simulink model "AirRefueling_Platform_PBVS"  (R2022b)
settings: Solver=ode4  StartTime=0.0  StopTime=60  FixedStep=0.01  RelTol=1e-5  AbsTol=1e-4  EnableMultiTasking=on
InitFcn:
  | F16_Init
values from neighbouring files (symbols this model uses):
  airSpeed = 393.72    [F16_Init.m]
  alpha0 = trimAlpha*180/pi    (= 6.62393794015)    [F16_Init.m]
  altitude = 9843    [F16_Init.m]
  b_ref = 30.0    (= 30)    [F16_Init.m]
  C = [ 1,0,0,zeros(1,15) ... (first row only)    [F16_Init.m]
  C2m = [C(1,:) ... (first row only)    [F16_Init.m]
  Cdr_ = 0.8    [hose_parameter4dock.mat]
  d_cam_rc = [4.7;0.54;-1.45] - [0;0;2.05]    [F16_Init.m]
  d_f_rc = [4.45;0;-3.81]    [F16_Init.m]
  d_pr_cam = d_pr_rc - d_cam_rc    [F16_Init.m]
  d_pr_rc = [8.2;0.45;-3.3]    [F16_Init.m]
  dLEF = 0    [F16_Init.m]
  dtheta10 = [0 0 0 0 0 0 0 0 0 0]    [hose_parameter4dock.mat]
  dtheta20 = [0 0 0 0 0 0 0 0 0 0]    [hose_parameter4dock.mat]
  fi_flag = 1    [F16_Init.m]
  height = 3000    [hose_parameter4dock.mat]
  k_reel = 0.5    [hose_parameter4dock.mat]
  Kc = [ ... (first row only)    [F16_Init.m]
  kd = 500    [hose_parameter4dock.mat]
  Ki = zeros(4,3)    [F16_Init.m]
  Kp = zeros(4,18)    [F16_Init.m]
  l0 = 1.44444444444    [hose_parameter4dock.mat]
  l1 = 2    [hose_parameter4dock.mat]
  l_density = 4.1    [hose_parameter4dock.mat]
  m0 = 5.92222222222    [hose_parameter4dock.mat]
  mass = 636.94    [F16_Init.m]
  Mdr = 29.5    [hose_parameter4dock.mat]
  N = 10    [hose_parameter4dock.mat]
  p0_rc = [-30.7;1;10]    [F16_Init.m]
  Rdr = 0.305    [hose_parameter4dock.mat]
  Rl = 0.0336    [hose_parameter4dock.mat]
  T_reel_initial = 1610    [hose_parameter4dock.mat]
  theta10 = [0.459903280115 0.432776206681 0.412025416789 0.390288667864 0.365355881715 0.340009787283 0.310854701374 0.281345523746 0.248396428993 0.214590627751]    [hose_parameter4dock.mat]
  theta20 = [0 0 0 0 0 0 0 0 0 0]    [hose_parameter4dock.mat]
  trim_ail = 0.00874607850103852    (= 0.00874607850104)    [F16_Init.m]
  trim_control = [trim_thrust;trim_ele;trim_ail;trim_rud]    [F16_Init.m]
  trim_ele = -2.97973164860638    (= -2.97973164861)    [F16_Init.m]
  trim_rud = 0.0680302158182712    (= 0.0680302158183)    [F16_Init.m]
  trim_state1 = [trim_state;0;0;0;0;0;0]    [F16_Init.m]
  trim_thrust = 2279.08519954656    (= 2279.08519955)    [F16_Init.m]
  visual_err = [0;0;0]    [F16_Init.m]
  vt0 = [120 0 0]    [hose_parameter4dock.mat]
undefined symbols (not defined in the file or in its folder): dockingPoint, F, MIL, STD
libraries: etargetslib x11, dspnetwork x10, aerolibconvert2 x6, aerolibasang x4, simulink x2, aerolibatmos2 x2, aerolibwind2 x2, aerolibobsolete x2, sharedtransform x2, aerolibutil x2, vrlib x1, aerolibadyn x1
(part 3 of 3)

== matlab function AirRefueling_Platform_PBVS/Hose-drogue system/MATLAB Function ==
  data: P_dr input; P_link10 input; P_hose_dr output
function P_hose_dr = fcn(P_dr,P_link10)
% P_link20=zeros(3,20);
% P_link20(:,1) = P_link10(:,1)/2;
% P_link20(:,2) = P_link10(:,1);
% P_link20(:,3) = (P_link10(:,2)+P_link10(:,1))/2;
% P_link20(:,4) = P_link10(:,2);
% P_link20(:,5) = (P_link10(:,3)+P_link10(:,2))/2;
% P_link20(:,6) = P_link10(:,3);
% P_link20(:,7) = (P_link10(:,4)+P_link10(:,3))/2;
% P_link20(:,8) = P_link10(:,4);
% P_link20(:,9) = (P_link10(:,5)+P_link10(:,4))/2;
% P_link20(:,10) = P_link10(:,5);
% P_link20(:,11) = (P_link10(:,6)+P_link10(:,5))/2;
% P_link20(:,12) = P_link10(:,6);
% P_link20(:,13) = (P_link10(:,7)+P_link10(:,6))/2;
% P_link20(:,14) = P_link10(:,7);
% P_link20(:,15) = (P_link10(:,8)+P_link10(:,7))/2;
% P_link20(:,16) = P_link10(:,8);
% P_link20(:,17) = (P_link10(:,9)+P_link10(:,8))/2;
% P_link20(:,18) = P_link10(:,9);
% P_link20(:,19) = (P_link10(:,10)+P_link10(:,9))/2;
% P_link20(:,20) = P_link10(:,10);
% %P_link20(:,20) = P_dr;
% P_link20_V60 = reshape(P_link20,60,1);


%% 

x = P_link10(1,:);
y = P_link10(2,:);
z = P_link10(3,:);
n=length(x)-1;% B样条曲线有n+1个控制点
k=4;% 三次B样条，因此阶数=次数+1

% 用于储存生成的点
X=[];
Y=[];
Z=[];

Nik_u=zeros(1,n+1);% 用于储存基函数
nodevector=U_quasi_uniform(n,k);% 生成节点向量

for u=0:0.01:1-0.01% 循环次数决定组成B样条曲线点的总数量
    for j=1:n+1% 生成Bi,3这一系列基函数
        Nik_u(j)=BaseFunction(j,k,u,nodevector);
    end
    % 由于B样条曲线具有局部支撑性，因此只有u周围一定区间会参与到计算
    X=[X,x*Nik_u'];
    Y=[Y,y*Nik_u'];
    Z=[Z,z*Nik_u'];
end
% 根据三次B样条插值的结果得到20根管子的位置
P_link20=zeros(3,20);
index = 1;
for i=1:length(X)/20:100
    P_link20(:,index)=[X(i),Y(i),Z(i)];
    index = index+1;
end

P_link20_V60 = reshape(P_link20,60,1);
% 再将锥套的真实位置传过去 此时是63*1(20根管子+1个锥套)的向量 前面60个是软管 最后三个是锥套
P_hose_dr = [P_link20_V60;P_dr];

== matlab function AirRefueling_Platform_PBVS/Hose-drogue system/DRdynamics/Hose-Drogue1/Calculate the External Force of the Links/MATLAB Function ==
  data: vr input; n input; Ref output; radius input; viscosity input; Cf output; Red output; Cd output; N parameter
function [Ref, Cf, Red, Cd] = C(vr,n,radius,viscosity, N)
% 计算雷诺数以及相应的摩擦系数Cf和压差系数Cd

% 单杆的速度、方向等用3*1的列向量表示
% vr = 连杆相对风速度 向量3*N
% n = 连杆的方向向量，想上为正 向量3*N
% viscosity  = 动粘度系数
% radius = 连杆半径

%——计算雷诺数———————————————————————————
cosa = zeros(1,N);
sina = zeros(1,N);
Ref = zeros(1,N);
Red = zeros(1,N);
for i = 1:N
    if norm(vr(:,i)) ~= 0
        cosa(i) = vr(:,i)'*n(:,i)/norm(vr(:,i));
        sina(i) = sqrt(1-cosa(i)^2);
        if sina(i) ~= 0
            Ref(i) = (pi*radius/viscosity)*norm(vr(:,i))/sina(i);
        else
            Ref(i) = 10^11;
        end
        Red(i) = norm(vr(:,i))*2*radius/viscosity;
    end
end

%——计算气动系数——————————————————————————
Cf = zeros(1,N);
Cd = zeros(1,N);
for i = 1:N
    %%%%Cf表%%%%%%%%%%%%%%%%%%%%%%%%
    if Ref(i)<=10^-2
        Cf(i) = 0;    %注意这里有改动
    elseif Ref(i)>10^-2 && Ref(i)<=10^4
        Cf(i) = 4.6409*Ref(i)^-0.6667;
    elseif Ref(i)>10^4 && Ref(i)<=10^10
        Cf(i) = 0.0464*Ref(i)^-0.1667;
    elseif Ref(i)>10^10
        Cf(i) = 0.001;
    end
    %%%%Cd表%%%%%%%%%%%%%%%%%%%%%%%%%
    if Red(i)<=10^-2
        Cd(i) = 0;   %注意这里有改动
    elseif Red(i)>10^-2 && Red(i)<=1
        Cd(i) = 10*Red(i)^-0.801;
    elseif Red(i)>1 && Red(i)<=180
        Cd(i) = 10*Red(i)^-0.4083;
    elseif Red(i)>180 && Red(i)<=4*10^5
        Cd(i) = 1.2;
    elseif Red(i)>4*10^5 && Red(i)<=4*10^6
        Cd(i) = 0.002128*Red(i)^0.3522;
    elseif Red(i)>4*10^6
        Cd(i) = 0.45;
    end
end

== matlab function AirRefueling_Platform_PBVS/Hose-drogue system/DRdynamics/Hose-Drogue1/Calculate the External Force of the Links/MATLAB Function1 ==
  data: vr input; Q output; n input; Cf input; Cd input; l1 input; density input; radius input; Rdr input; Cdr input; Mdr input; rou input; p input; Fb input; Df_mid output; Dd_mid output; Df output; Dd output; D output; Ddr output; N parameter; l0 parameter; fen_norm output; fen output
function [Q, Df_mid, Dd_mid, Df, Dd, D, Ddr, fen_norm, fen] = ExternalForce(vr,n,Cf,Cd,l1,density,radius,Rdr,Cdr,Mdr,rou,p,Fb, N,l0)

% 计算每根连杆的合外力

% 单杆的速度、方向等用3*1的列向量表示
% l = 每根连杆的长度，注意这里要做成变长的 向量
% vr = 连杆相对风速度 向量3*N
% n = 连杆的方向向量，想上为正 向量3*N
% viscosity  = 大气动粘度系数
% density = 大气密度
% radius = 连杆半径
% r_dr = 锥套伞冠半径
% rou = 连杆的线密度

% Cdr = 锥套的阻力系数
% Rdr = 锥套伞冠半径
% Mdr = 锥套质量

%——求气动力————————————————————————————
Df_mid = zeros(1,N);
Dd_mid = zeros(1,N);
Df = zeros(3,N);
Dd = zeros(3,N);
D = zeros(3,N);
vn = zeros(3,N);
for i = 1:N
    if i == 1
        Df_mid(i) = density*pi*radius*l1*Cf(i)*(vr(:,i)'*n(:,i))^2;
    else
        Df_mid(i) = density*pi*radius*l0*Cf(i)*(vr(:,i)'*n(:,i))^2;
    end
    if vr(:,i)'*n(:,i)>0   % 这里可能有符号问题，万一之后还是出现杂乱的情况，要注意这里
        Df(:,i) = Df_mid(i)*n(:,i);
    else
        Df(:,i) = - Df_mid(i)*n(:,i);
    end
    % 当杆的方向迎着风的时候，摩擦阻力延杆反向
    % 当杆的方向顺着风的时候，摩擦阻力延杆正向
    
    vn(:,i) = vr(:,i)-(vr(:,i)'*n(:,i))*n(:,i); 
    if i == 1
        if norm(vn(:,i)) ~= 0
            Dd_mid(i) = density*radius*l1*Cd(i)*norm(vn(:,i))^2;
            Dd(:,i) = - Dd_mid(i)*vn(:,i)/norm(vn(:,i));
        else
            Dd(:,i) = [0;0;0];
        end
    else
        if norm(vn(:,i)) ~= 0
            Dd_mid(i) = density*radius*l0*Cd(i)*norm(vn(:,i))^2;
            Dd(:,i) = - Dd_mid(i)*vn(:,i)/norm(vn(:,i));
        else
            Dd(:,i) = [0;0;0];
        end
    end
    % 无论连杆与相对速度的角度关系如何，压差阻力总是顺着风的方向的
        
    D(:,i) = Df(:,i) + Dd(:,i);
end

if vr(:,N)'*vr(:,N) ~= 0
    Ddr = - 1/2*density*vr(:,N)'*vr(:,N)*(pi*Rdr^2)*(Cdr)* vr(:,N)/norm(vr(:,N));
else
    Ddr = [0;0;0];
end
%%%%%%%%%%%%%%%%%%%%%%%%%%%%%%%%%%%%%%%%%%%%%%%%%%%%%%%%%%%%%%%%

% %%%%计算恢复力%%%%%%%%%%%%%%%%%%%%%%
do = 1; % 连杆外径
di = 0.84; % 连杆内径
E = 589.67; % 弹性系数 数量级可能有问题
K = E*pi/8*(do^4 - di^4);
fen_norm = zeros(1,N);
fen = zeros(3,N);
for i = 2:N-1
    n0mid = (p(:,i-1) - p(:,i+1))/norm(p(:,i-1) - p(:,i+1));
    if abs(norm(n(:,i-1)'*n(:,i))-1) ~= 0;
        gama1 = n(:,i-1)'*n0mid;
        gama2 = n(:,i)'*n0mid;
        if norm(gama1) >= 1
            gama1 = gama1/abs(gama1);
        end
        if norm(gama2) >= 1
            gama2 = gama2/abs(gama2);
        end
            
        fen_norm(i) = K*(acos(gama1) + acos(gama2))/norm(p(:,i-1) - p(:,i+1))^2;
        fen(:,i) = fen_norm(i)*((n(:,i)'*n0mid*n0mid - n(:,i))*1e3)/norm((n(:,i)'*n0mid*n0mid - n(:,i))*1e3);
    end
end
%%%%%%%%%%%%%%%%%%%%%%%%%%%%%%%%%%%%%%

% %%%%计算合外力%%%%%%%%%%%%%%%%%%%%%%?
% Q = zeros(3,N);
% for i = 1:N-1
%     Q(:,i) = [0;0;m*g] + 1/2*(D(:,i)+D(:,i+1));
% end
% Q(:,N) = [0;0;(m+Mdr)*g] + 1/2*D(:,N) + Ddr;
Q = zeros(3,N);
Q(:,1) = [0;0;l1*rou*9.8] + 1/2*(D(:,1)+D(:,2)) + fen(:,1);
for i = 2:N-1
    Q(:,i) = [0;0;l0*rou*9.8] + 1/2*(D(:,i)+D(:,i+1)) + fen(:,i);
end
Q(:,N) = [0;0;(l0/2*rou + Mdr)*9.8] + 1/2*D(:,N) + Ddr + Fb;        %注意最后一个节点的质量
% 这里删掉了锥套的受力（Bow wave），后面再处理
% %%%%%%%%%%%%%%%%%%%%%%%%%%%%%%%%

== matlab function AirRefueling_Platform_PBVS/Hose-drogue system/DRdynamics/Hose-Drogue1/Calculate the Orientation of the Links1/MATLAB Function ==
  data: nd1 output; nd2 output; theta1 input; n output; theta2 input; N parameter
function [nd1,nd2,n] = fcn(theta1,theta2, N)
% theta1,theta2 向量1*n
n = zeros(3,N);
nd1 = zeros(3,N);
nd2 = zeros(3,N);

for i = 1:N
    n(:,i) = [cos(theta1(i))*cos(theta2(i)); sin(theta2(i)); -sin(theta1(i))*cos(theta2(i))];
    nd1(:,i) = [-sin(theta1(i))*cos(theta2(i)); 0; -cos(theta1(i))*cos(theta2(i))];
    nd2(:,i) = [-cos(theta1(i))*sin(theta2(i)); cos(theta2(i)); sin(theta1(i))*sin(theta2(i))];
end

== matlab function AirRefueling_Platform_PBVS/Hose-drogue system/DRdynamics/Hose-Drogue1/Calculate the Orientation of the Links1/MATLAB Function4 ==
  data: a input; a0 input; nd1 input; nd2 input; dn input; dnd1 input; dnd2 input; dtheta1 input; dtheta2 input; l1 input size=1; dl1 input; ddtheta1 output; ddtheta2 output; N parameter; l0 parameter
function [ddtheta1,ddtheta2] = fcn(a,a0,nd1,nd2,dn,dnd1,dnd2,dtheta1,dtheta2,l1,dl1, N, l0)
% theta1,theta2 向量N*1
% omiga,alpha是加油机坐标系的旋转角速度和叫加速度
% a是各节点的加速度
% a0为加油机加速度
% l,dl,ddl是连杆的长度及其一二阶导数

ddtheta1 = zeros(1,N);
ddtheta2 = zeros(1,N);

ddtheta1(1) = nd1(:,1)'*(-(a(:,1)-a0)-2*dl1*dn(:,1)-...
              l1*(dnd1(:,1)*dtheta1(1)+dnd2(:,1)*dtheta2(1)))...
              /(l1*norm(nd1(:,1)));
ddtheta2(1) = nd2(:,1)'*(-(a(:,1)-a0)-2*dl1*dn(:,1)-...
              l1*(dnd1(:,1)*dtheta1(1)+dnd2(:,1)*dtheta2(1)))...
              /(l1*norm(nd2(:,1)));
for i = 2:N
    ddtheta1(i) = nd1(:,i)'*(-(a(:,i)-a(:,i-1))-...
                  l0*(dnd1(:,i)*dtheta1(i)+dnd2(:,i)*dtheta2(i)))...
                  /(l0*norm(nd1(:,i)));
    ddtheta2(i) = nd2(:,i)'*(-(a(:,i)-a(:,i-1))-...
                  l0*(dnd1(:,i)*dtheta1(i)+dnd2(:,i)*dtheta2(i)))...
                  /(l0*norm(nd2(:,i)));
end

== matlab function AirRefueling_Platform_PBVS/Hose-drogue system/DRdynamics/Hose-Drogue1/Calculate the Orientation of the Links1/MATLAB Function5 ==
  data: v0 input; n input; dn input; l1 input; dl1 input; w input; vr output; p0 input; p output; N parameter; l0 parameter; pdr output
function [vr,p,pdr] = fcn(v0,n,dn,l1,dl1,w,p0, N, l0)

% v0为加油机速度
% l,dl是连杆的长度及其一阶导数
% wt为合成风在每个节点的风速
% p0为预留，在计算相对地面的位置时用到

vr = zeros(3,N);
vr(:,1) = v0 - dl1*n(:,1) - l1*dn(:,1) ;
for i = 2:N
    vr(:,i) = vr(:,i-1) - l0*dn(:,i);
end
vr = vr - w;

p = zeros(3,N);
p(:,1) = [0;0;0] - l1*n(:,1);
for i = 2:N
    p(:,i) = p(:,i-1) - l0*n(:,i);
end
pdr = p(:,N) + [-0.3;0;0];
% pdr = p(:,N);

== matlab function AirRefueling_Platform_PBVS/Receiver system/Guidance ==
  settings: updateMethod=DISCRETE
  data: dd input; estimate_dr2pr input; y output; t input; d_x output; t_d output
function [y,d_x,t_d] = fcn(dd,estimate_dr2pr,t)
%#codegen
%dd是锥管前端位置，dx是锥套位置（dx输入前第三分量换号，已由x,y,h转化为x,y,z）
%dx输入前减去常数：控制中控制的是受油机质心而非锥管前端，所以参考轨迹也要由锥管的参考轨迹转化为受油机质心的参考轨迹。
%控制的目的就是最终令dd和dx相等，让受油机质心跟踪参考位置

% y=dx; 输出y的意思是让受油机飞行的三维距离，和之前初始化定义受油机三维位置不同
%% 理想的对接点是  [9.5100;-1.4550;-0.0830]+[0.2;0;0] 9.5m时是第一节探头进锥套 最多再多0.2m此时是第一节抵住中间小黑圈
persistent aa;
if(isempty(aa))   %%aa(1:3)为锥套平衡位置,(4:6)为锥套实际位置或其滤波位置，(7:9)是锥管实际位置或其滤波位置；
    aa=zeros(9,1);
end

% 这个tt是用来对总体的时间逻辑进行控制的
persistent tt;
if(isempty(tt))
    tt=0;
end
% 这个t_dock是用来记录对接成功的初始时间的，这样就能
persistent t_dock;
if(isempty(t_dock))
    t_dock=0;
end
t_d=t_dock;

% 这个t_lock是用来锁定对接时间的，标识为1时说明已经锁定了对接时间
persistent t_lock;
if(isempty(t_lock))
    t_lock=0;
end

% 判断是否可以脱离对接，再进行下一次的对接
persistent flag_can_dock;
if(isempty(flag_can_dock))
    flag_can_dock=1;
end

persistent nn;    %%nn为前馈量
if(isempty(nn))
    nn=[0;0;0];
end

persistent dx;     %%锥套位置距离其平衡位置的偏差
if(isempty(dx))
    dx=[0;0;0];
end
d_x=dx;

% 使用额外飞行的距离来对碰撞模块和HDU进行验证
extra_flight=[0.5;0;0];
%% y为期望轨迹
% tt是上次对接成功时候记录的时间
t1=t-tt;
if t1<20
    y=[8;-1.8;0.4];
    aa(1:3)=y;
elseif t1<30
    y = aa(1:3);
    if t1>24 && t1<25
        % 此时的aa(1:3)约等于[8;-1.8;0.4]，estimate_pr2dt=[1.61;0.345;-0.483]
        dx = aa(1:3)+ estimate_dr2pr;
    end
    if t1>25
        dx(1:3) = 3/4 * dx(1:3) + 1/4 * (aa(1:3) + estimate_dr2pr);
    end
else   
    y = [dx(1)+nn(1);dx(2)+nn(2);dx(3)+nn(3)]+extra_flight ; 
%     y = 0.5 * ([dx(1)+nn(1);dx(2)+nn(2);dx(3)+nn(3)]+[dx(1)+dd(1);dx(2)+dd(2);dx(3)+dd(3)]);     
%%  这里是近距离对接过程的判断
    if abs(dd(1)-dx(1))<0.01 && flag_can_dock == 1  % 状态为可以对接 且 锥管锥套距离达到对接要求 认为是一次对接
       % 认为已经对接上了 所以标志位要清零, 同时记录对接的时间t_dock
       flag_can_dock = 0;
       t_lock = 1;
       if(t_lock == 1 && flag_can_dock == 0)
           % 在对接成功时，虽然满足0.01的条件，但是不满足后面==1的条件 所以对接时间不会多次记录
          t_dock = t;
       end
    end
    
   % t_dock保存的就是对接成功的时间 当保持的时间大于20s时，才进行下一次对接
   % 在对接状态 且 持续时间超过了10s 就设置为脱离状态
   if(t-t_dock>=10 && flag_can_dock == 0 )
       flag_can_dock=1;
           % 如果对接的时间到 那么锥套椎管放开接触 标志位置1，意味着可以对接
       if(flag_can_dock == 1)
           % 更新前馈量 aa(4:6)存储的是锥套的滤波位置 aa(7:9)存储的是椎管的滤波位置
           nn=nn+[0.6*sat((aa(4)-aa(7))/0.6);0.6*sat((aa(5)-aa(8))/0.6);0.6*sat((aa(6)-aa(9))/0.6)];

           % 省去了前面的过程  时间如果一减掉 调用脚本的时候就跳出这个代码范围 相当于回到第10s时候的状态
           tt=t-10;
       end   
   end    
          
    % 当距离小于0.4m的时候，进行滤波
    if abs(dd(1)-dx(1))<0.4 && flag_can_dock == 1
        aa(4:6)=2/3 * aa(4:6)+ 1/3 * dx;
        aa(7:9)=2/3 * aa(7:9)+ 1/3 * dd;
    end  
    % 当小于0.5m大于0.4m的时候，记录位置
    if abs(dd(1)-dx(1))<0.5 && flag_can_dock == 1
        aa(4:6)=dx;
        aa(7:9)=dd;
    end 
end

== matlab function AirRefueling_Platform_PBVS/Hose-drogue system/DRdynamics/Hose-Drogue1/MATLAB Function3 ==
  data: n input; alpha output; N parameter
function alpha = fcn(n, N)
% 计算两杆之间的弯折角度，用来粗略的验证恢复力的效果
alpha = zeros(1,N);
for i = 2:N
    mid = n(:,i-1)'*n(:,i);
    if abs(mid) > 1
        mid = mid/abs(mid);
    end
    alpha(i) = acos(mid)/pi*180;
end

== matlab function AirRefueling_Platform_PBVS/Visual process/VehicleDataParse ==
  data: Data input; CopterID output; Length input; Out output; checksum input; len input
function [CopterID,Out] = fcn(Data,Length,checksum,len)

% 设定静态变量，在数据校验失败时，保持上一时刻值
persistent DataOut;
if isempty(DataOut)
    DataOut=zeros(16,1);
end
persistent cpID;
if isempty(cpID)
    cpID=0;
end

% 如果包长不等于设定值，这个包丢弃，使用原来的值
if Length ~= len %如果包长度不匹配，校验不通过，那么使用上一时刻值
    Out=DataOut;
    CopterID=cpID;
    return;
end

CkSum = typecast(Data(1:4), 'int32');
if CkSum ~= checksum %如果校验码不匹配，校验不通过，那么使用上一时刻值
    Out=DataOut;
    CopterID=cpID;
    return;    
end

% 提取数据
CpIDTmp = typecast(Data(5:8), 'int32');
DataTmp = typecast(Data(9:136), 'double');
% DataTmp=zeros(16,1);
for i=1:16
    idx = (i-1)*8+9;
    DataTmp(i) = typecast(Data(idx:idx+7), 'double');
end



% 配置输出数据
CopterID = double(CpIDTmp);
Out = DataTmp;

% 记录上一时刻值
cpID=CopterID;
DataOut=Out;

== matlab function AirRefueling_Platform_PBVS/SimToUE11 ==
  data: y output; PosPr1 input; PosTb1 input
function y = SimToVR(PosPr1,PosTb1)
%#codegen

%%函数名：SimToVR
%%用途  ：将软管锥套坐标输出转换为VR输入
%%输入  ：PosPr - 受油机椎管坐标， PlsTb - 软管坐标数据
%%输出  ：VrPos - 软管和受油机VR位置，VrAngle - 旋转角度输出
%%作者  ：戴训华
%%时间  ：2014/3/19

%{
PosPr = PosPr1(1:3);
% add PosPr1(4:6)存储的是受油机的姿态  模型中在输出姿态[phi, theta, psai]后加上了trim_state1=[0;0.1156,0],这里又给减掉了
% 无人机先绕机体系 z 轴旋转 ψ \psiψ，再绕机体系 y 轴旋转 θ \thetaθ，最后绕机体系 x 轴旋转 ϕ \phiϕ，[yaw,pitch,roll]
% AttitudeRecei = [PosPr1(4);-PosPr1(6);PosPr1(5)-0.115609];
AttitudeRecei = [PosPr1(4);-PosPr1(6);PosPr1(5)-0.115609];
PosTb = PosTb1(1:60);
% 这里是20根软管+1个锥套+1个受油机 
VrAngle = zeros(22*3,1);
VrPos = zeros(22*3,1);
% add
scale = 1;
for j = 1:21                        %前20为软管坐标数据，后1为软管平滑过渡处理
    if j == 1
        pX = [0, 0, 0]';            %软管起点
        pY = PosTb(3*j-2:3*j);      %软杆终点
    elseif j == 21                  %多加一段杆，做过渡
        pX = PosTb(3*j-5:3*j-3);
        pY = [PosTb(3*j-5)-0.7163*cos(8/180*pi),PosTb(3*j-4),PosTb(3*j-3)+0.7163*sin(8/180*pi)]';
    else
        pX = PosTb(3*j-5:3*j-3);
        pY = PosTb(3*j-2:3*j); 
    end
    
    pZ = (pX + pY)/2;               %中点坐标
    if j==21
        % 给一个锥套的偏置
        pZ = pZ + [0,0,-0.25]';
    end
%     pZ = pZ * 8/3;                  %到VR中比例的缩放
    pZ = pZ * scale;
    
    vAxis = [0,0,-1]';               %水平轴
    vTb = pY - pX;                  %杆的方向
    
    axis1 = null([vAxis';vTb']);%获取垂直向量
    vRot = axis1(:,1)';             %得到旋转轴
    
    if vRot(2) < 0
        vRot = -vRot;
    end
 
    yaw_xoz = asin(vTb(2) / sqrt(vTb(1)*vTb(1) + vTb(2)*vTb(2)+ vTb(3)*vTb(3)));
    pitch_z = pi - atan(vTb(3) / vTb(1));
%     pitch_z = atan(vTb(3) / vTb(1));
    roll = 0;   % 圆柱形hose，不用计算roll   
    VrAngle(3*j-2:3*j) = [yaw_xoz, pitch_z, roll];
    VrPos(3*j-2:3*j) = [pZ(1),pZ(2),pZ(3)]';
end
%y = u;
% add 发送的是受油机的位置
VrAngle(64:66)=[AttitudeRecei(1);AttitudeRecei(2);AttitudeRecei(3)];
% add PosPr(1:3)受油机椎管的坐标  [0 -0.1 -0.05]'是椎管相对于受油机的位置
pZ = PosPr+[0 -0.1 -0.05]';
pZ = pZ * scale;
% pZ = pZ * 8/3;
% 旋转坐标系
VrPos(3*22-2:3*22) = [pZ(1),pZ(2),pZ(3)]';
tmp1 = VrPos(1:60,:); % 软管位置
% delta_drogue =[0 0 0.5]'; 
delta_drogue =[-0.8 0 0.45]'; 
% delta_drogue =[-0.2 0 0.3]'; 
tmp2 = VrPos(61:63,:)+ delta_drogue;% 锥套位置
tmp3 = VrPos(64:66,:);% 受油机位置
tmp4 = VrAngle(1:60,:); % 软管角度
tmp5 = VrAngle(61:63,:)+[0 0.09 0]';% 锥套角度
tmp6 = VrAngle(64:66,:);% 受油机角度
tmp=[tmp1;tmp4;tmp2;tmp5;tmp3;tmp6];
y = tmp;
%}

%%
%%函数名：SimToVR
%%用途  ：将软管锥套坐标输出转换为VR输入
%%输入  ：PosPr - 受油机椎管坐标， PlsTb - 软管坐标数据 60*1 10根管子的位置（每根管子的中心位置和尾部位置，一共10*3+10*3=60个数据） 
%%输出  ：VrPos - 软管和受油机VR位置，VrAngle - 旋转角度输出

PosPr = PosPr1(1:3);
% add PosPr1(4:6)存储的是受油机的姿态  模型中在输出姿态[phi, theta, psai]后加上了trim_state1=[0;0.1156,0],这里又给减掉了
% 无人机先绕机体系 z 轴旋转 ψ \psiψ，再绕机体系 y 轴旋转 θ \thetaθ，最后绕机体系 x 轴旋转 ϕ \phiϕ，[yaw,pitch,roll]
% AttitudeRecei = [PosPr1(4);-PosPr1(6);PosPr1(5)-0.115609];
% AttitudeRecei = [PosPr1(4);PosPr1(5);PosPr1(6)];
AttitudeRecei = [0;0.1156;0];
%% 这个模型中是10个软管，传入的60*1的数组中，已经包含了杆子中心的坐标
PosTb = PosTb1(1:60);
% 这里是10根软管+1个锥套+1个受油机,全部是列向量
VrAngle = zeros(12*3,1);
VrPos = zeros(12*3,1);
% add
scale = 1;
for j = 1:11                                        %10根为软管坐标数据 第11根为锥套的坐标数据
    if j == 11                                      %多加一段杆，做过渡
        pX = PosTb(6*(j-1)-2:6*(j-1));              %选择最后一个位置作为锥套的pX
        pY = [PosTb(6*(j-1)-2)-0.7163*cos(8/180*pi),PosTb(6*(j-1)-1),PosTb(6*(j-1))+0.7163*sin(8/180*pi)]';     % 这个位置是平滑出来的，用作方向,大概是虚拟的第11根杆的中点
        pZ = pY + [0,0,0]';
    else
        pX = PosTb(6*(j-1)+1:6*(j-1)+3);            %第一根软管的中点，起点是(0,0,0)
        pY = PosTb(6*(j-1)+4:6*(j-1)+6);            %软杆终点
        pZ = pX;                                    %中点坐标，前面的程序中计算过了，直接赋值
    end
    pZ = pZ * scale;
    vAxis = [0,0,-1]';               %水平轴
    vTb = pY - pX;                  %杆的方向
    
    axis1 = null([vAxis';vTb']);%获取垂直向量
    vRot = axis1(:,1)';             %得到旋转轴
    
    if vRot(2) < 0
        vRot = -vRot;
    end
 
    yaw_xoz = asin(vTb(2) / sqrt(vTb(1)*vTb(1) + vTb(2)*vTb(2)+ vTb(3)*vTb(3)));
    pitch_z = pi - atan(vTb(3) / vTb(1));
%     pitch_z = atan(vTb(3) / vTb(1));
    roll = 0;   % 圆柱形hose，不用计算roll   
    VrAngle(3*j-2:3*j) = [yaw_xoz, pitch_z, roll];
    VrPos(3*j-2:3*j) = [pZ(1),pZ(2),pZ(3)]'+[0,0,-1]';
end
%y = u;
% add 发送的是受油机的姿态
VrAngle(34:36)=[AttitudeRecei(1);AttitudeRecei(2);AttitudeRecei(3)];
% add PosPr(1:3)受油机椎管的坐标  [0 -0.1 -0.05]'是微调椎管相对于受油机的位置
pZ = PosPr+[0 -0.1 -0.05]';
pZ = pZ * scale;
VrPos(34:36) = [pZ(1),pZ(2),pZ(3)]';

tmp1 = VrPos(1:30); % 软管位置
% delta_drogue_pos =[-0.8 0 0.45]'; 
% delta_drogue_atti=[0 0.09 0]';
delta_drogue_pos =[0 0 0]'; 
delta_drogue_atti=[0 0.09 0]';
tmp2 = VrPos(31:33)+ delta_drogue_pos;% 锥套位置
tmp3 = VrPos(34:36);% 受油机位置
tmp4 = VrAngle(1:30); % 软管角度
tmp5 = VrAngle(31:33)+delta_drogue_atti;% 锥套角度
tmp6 = VrAngle(34:36);% 受油机角度
tmp=[tmp1;tmp4;tmp2;tmp5;tmp3;tmp6];
y = tmp;

== matlab function AirRefueling_Platform_PBVS/Hose-drogue system/DRdynamics/Hose-Drogue1/Calculate the Acceleration of the Links1/MATLAB Function ==
  data: n input; m1 input; T output; m0 parameter; N parameter
function T = fcn(n,m1, m0,N)

% n = 连杆的方向向量，想上为正 向量3*N
% m = 连杆的质量 向量1*N

%%%%求张力t%%%%%%%%%%%%%%%%%%%%%%%%%%%%%%%%%%%%%%%%%%%%%%%%%%%%%%
T = zeros(N,N);

T(1,1) = 1;
T(1,2) = - n(:,1)'*n(:,2);
T(N,N-1) = -1/m0*n(:,N-1)'*n(:,N);
T(N,N) = 1/m0 + 1/m0;             %注意这里很重要！！

T(2,1) = -1/m1*n(:,1)'*n(:,2);
T(2,2) = 1/m1 + 1/m0;
T(2,3) = -1/m0*n(:,2)'*n(:,3);

for i = 3:N-1
    T(i,i-1) = -1/m0*n(:,i-1)'*n(:,i);
    T(i,i) = 1/m0 + 1/m0;
    T(i,i+1) = -1/m0*n(:,i)'*n(:,i+1);
end

== matlab function AirRefueling_Platform_PBVS/Tanker system/  ==
  data: u input; y output

function y = WindTurFromTank(u)
%#codegen

%横纵向气流角速度等下计算长度
c_lat=4;
c_lon=4;

%两端参考点
u1 = u+[0 ,c_lat ,0]';
u2 = u+[0 ,-c_lat, 0]';

yy1 = TankerVortexWindField(u1);
yy2 = TankerVortexWindField(u2);

%计算x轴向滚转角速度
yp = (yy1(3) - yy2(3))/4/c_lat;

u3=u+[c_lon, 0,0]';
u4=u+[-c_lon ,0,0]';
yy3 = TankerVortexWindField(u3);
yy4 = TankerVortexWindField(u4);

%俯仰角速度计算
yq = -(yy3(3) - yy4(3))/4/c_lon;

%偏航角速度设为0
yr = 0;

%质心处风场计算
y_uvw = TankerVortexWindField(u);


%y = [y_uvw(1);y_uvw(2);y_uvw(3);-yp;-yq;-yr]*0.5;
y = [y_uvw(1);y_uvw(2);y_uvw(3);-yp;-yq;-yr];

== matlab function AirRefueling_Platform_PBVS/SimToVR1 ==
  data: PosPr1 input; PosTb1 input; y output
function y = SimToVR(PosPr1,PosTb1)
%#codegen

%%函数名：SimToVR
%%用途  ：将软管锥套坐标输出转换为VR输入
%%输入  ：PosPr - 受油机椎管坐标， PlsTb - 软管坐标数据
%%输出  ：VrPos - 软管和受油机VR位置，VrAngle - 旋转角度输出
%%作者  ：戴训华
%%时间  ：2014/3/19

PosPr = PosPr1(1:3);
AttitudeRecei = [0;-0;0+0.115609];

PosTb = PosTb1(1:60);

VrAngle = zeros(22*4,1);
VrPos = zeros(22*3,1);


for j = 1:21                        %前20为软管坐标数据，后1为软管平滑过渡处理
    if j == 1
        pX = [0, 0, 0]';            %软管起点
        pY = PosTb(3*j-2:3*j);      %软杆终点
    elseif j == 21                  %多加一段杆，做过渡
        pX = PosTb(3*j-5:3*j-3);
        pY = [PosTb(3*j-5)-0.7163*cos(8/180*pi),PosTb(3*j-4),PosTb(3*j-3)+0.7163*sin(8/180*pi)]'+[0;-0.2;0];
    else
        pX = PosTb(3*j-5:3*j-3);
        pY = PosTb(3*j-2:3*j); 
    end
    
    pZ = (pX + pY)/2;               %中点坐标
    pZ = pZ * 8/3;                  %到VR中比例的缩放

    vAxis = [0,0,-1]';               %水平轴
    vTb = pY - pX;                  %杆的方向
    
    axis1 = null([vAxis';vTb']);%获取垂直向量
    vRot = axis1(:,1)';             %得到旋转轴
    
    if vRot(2) < 0
        vRot = -vRot;
    end
    
    VrAngle(4*j-3:4*j-1) = [vRot(1),vRot(3),vRot(2)]';
    VrAngle(4*j) = acos(vAxis'*vTb / sqrt(vAxis'*vAxis * vTb'*vTb));
    
    VrPos(3*j-2:3*j) = [pZ(1),-pZ(3),pZ(2)]';
end
%y = u;
VrAngle(81:84)=VrAngle(81:84)+[0.2714;0;0;0]; %微调锥套姿态
VrPos(61:63)=VrPos(61:63)+[0;0.00;0.25];      %微调锥套位置

VrAngle(85:88)=[AttitudeRecei(1);AttitudeRecei(2);AttitudeRecei(3);norm(AttitudeRecei)];
pZ = PosPr+[0 0-0.1 0-0.1]';
pZ = pZ * 8/3;
VrPos(3*22-2:3*22) = [pZ(1),-pZ(3),pZ(2)]';

y = [VrAngle;VrPos];

== matlab function AirRefueling_Platform_PBVS/Hose-drogue system/DRdynamics/HDU/MATLAB Function1 ==
  data: l1 input; l1initial input; dl1 input; flag1 output size=1; l1out output; dl1out output; ddl1 input; ddl1out output
function [flag1,l1out,dl1out,ddl1out] = fcn(l1,l1initial,dl1,ddl1)
% 如果第一根管子的长度比初始值大 或者 第一根管子的加速度>0 那么就是要控制了 flag从0变1开始积分
if (l1 > l1initial) || (l1 == l1initial && dl1 > 0)
    flag1 = 1;
    l1out = l1initial;
    dl1out = 0;
    ddl1out = 0;
else
    flag1 = 0;
    l1out = l1;
    dl1out = dl1;
    ddl1out = ddl1;
end

== matlab function AirRefueling_Platform_PBVS/Hose-drogue system/Bow Wave Effect/Bow Wave Effect Function ==
  data: x input; Fx output; y input; z input; Fy output; Fz output
function [Fx,Fy,Fz] = F_rc2dr(x,y,z)
Cx1 = 91.6170;
Cx2 = 0.3220;
Cx3 = 3.8870;
Cx4 = 2.7359;
Cx5 = 2.4939;
Cx6 = 309.7709;
Cx7 = 0.3237;
Cx8 = 0.3851;
Cx9 = 1.1471;

Cy1 = 223.3210;
Cy2 = 0.2082;
Cy3 = 0.8102;
Cy4 = 0.6555;

Cz1 = 173.2021;
Cz2 = 0.2141;
Cz3 = 0.5697;
Cz4 = 0.7038;

if x > 5.6493
    Fx = 0;
elseif x > 3.0893
    Fx = Cx1*(1-Cx2*(x-Cx3)^2)*exp(-y^2/Cx4)*exp(z/Cx5);
else
    Fx = Cx1*(1-Cx2*(x-Cx3)^2)*exp(-y^2/Cx4)*exp(z/Cx5)...
       + Cx6*(1-Cx7*x)*exp(-y^2/Cx8)*exp(z/Cx9);
end

if x > 4.8031
    Fy = 0;
else
    Fy = Cy1*(1-Cy2*x)*(y*exp(-y^2/Cy3))*exp(z/Cy4);
end

if x > 4.6275
    Fz = 0;
else
    Fz = -Cz1*(1-Cz2*x)*exp(-y^2/Cz3)*exp(z/Cz4);
end

== matlab function AirRefueling_Platform_PBVS/Hose-drogue system/Total Turbulence   ==
  data: u1 input; u input; y output
function y = Dr_wind2Frc(u1,u)
%#codegen

Ve=120;
rho = 0.98;
Q=0.5*rho*Ve^2;
S=0.38;
CD=0.81*0.8;

uu=u(1);
vv=u(2);
ww=u(3);

%beta = acos(sqrt(vv^2+ww^2)/abs(uu));
%theta = atan(ww/vv);

C_beta = 0.3979;

yx=rho*S*CD*Ve*uu;
yy=Q*S*C_beta*vv/Ve;
yz=Q*S*C_beta*ww/Ve;

% 这个y_v是有涡流+自然风所得到的速度换算成的位置偏移
y_v = [yx,yy,yz]';
y=[y_v;u1+y_v];
